simulink model "Sensores"  (R2023b)
settings: Solver=VariableStepAuto  StartTime=0.0  StopTime=10.0  RelTol=1e-3
undefined symbols (not defined in the file): magnitude, Tau_sens_temp, w_n_sens_corr, w_n_sens_pos, zeta_sens
settings Model: Creator=tomas  LastModifiedBy=tomas

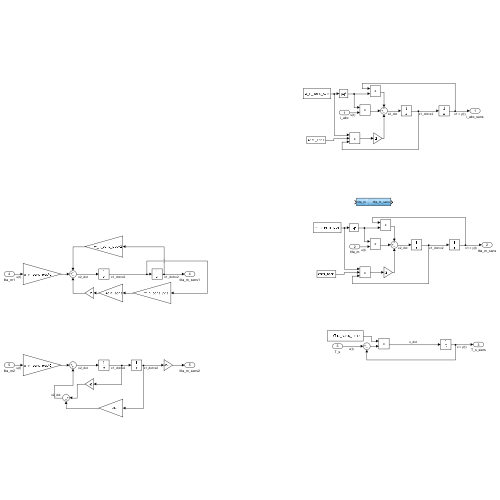
[thumbnail: Simulink's stored preview of the top-level diagram]
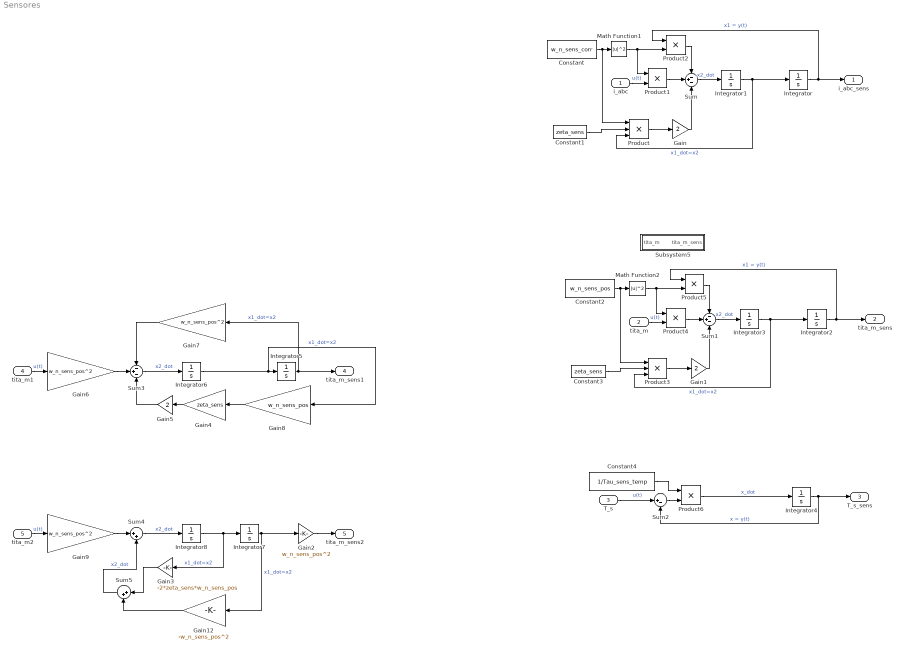
== system Sensores ==
  i_abc : Inport
  tita_m : Inport  Port=2
  T_s : Inport  Port=3
  tita_m1 : Inport  Port=4
  tita_m2 : Inport  Port=5
  Constant : Constant  Value=w_n_sens_corr
  Constant1 : Constant  Value=zeta_sens
  Constant2 : Constant  Value=w_n_sens_pos
  Constant3 : Constant  Value=zeta_sens
  Constant4 : Constant  Value=1/Tau_sens_temp
  Gain : Gain  Gain=2
  Gain1 : Gain  Gain=2
  Gain12 : Gain  Gain=-w_n_sens_pos^2
  Gain{2,6..7,9} (4 alike) : Gain  Gain=w_n_sens_pos^2
  Gain3 : Gain  Gain=-2*zeta_sens*w_n_sens_pos
  Gain4 : Gain  Gain=zeta_sens
  Gain5 : Gain  Gain=2
  Gain8 : Gain  Gain=w_n_sens_pos
  Integrator{,1..8} (9 alike) : Integrator
  Math Function1 : Math  Operator=magnitude^2
  Math Function2 : Math  Operator=magnitude^2
  Product : Product  Inputs=3
  Product{1..2,4..6} (5 alike) : Product
  Product3 : Product  Inputs=3
  Subsystem5 : Subsystem
  Sum : Sum  Inputs=-+-
  Sum1 : Sum  Inputs=-+-
  Sum2 : Sum  Inputs=|+-
  Sum3 : Sum  Inputs=-+-
  Sum4 : Sum  Inputs=|++
  Sum5 : Sum  Inputs=|++
  i_abc_sens : Outport
  tita_m_sens : Outport  Port=2
  T_s_sens : Outport  Port=3
  tita_m_sens1 : Outport  Port=4
  tita_m_sens2 : Outport  Port=5
  wires:
  Integrator/1 -> i_abc_sens/1, Product2/1  "x1 = y(t)"
  Integrator1/1 -> Product/3, Integrator/1  "x1_dot=x2"
  Constant/1 -> Product/1, Math Function1/1
  i_abc/1 -> Product1/2  "u(t)"
  Math Function1/1 -> Product2/2, Product1/1
  Product1/1 -> Sum/2
  Product2/1 -> Sum/1
  Product/1 -> Gain/1
  Gain/1 -> Sum/3
  Sum/1 -> Integrator1/1  "x2_dot"
  Constant1/1 -> Product/2
  Product4/1 -> Sum1/2
  Gain1/1 -> Sum1/3
  Constant2/1 -> Product3/1, Math Function2/1
  tita_m/1 -> Product4/2  "u(t)"
  Product3/1 -> Gain1/1
  Product5/1 -> Sum1/1
  Math Function2/1 -> Product5/2, Product4/1
  Sum1/1 -> Integrator3/1  "x2_dot"
  Constant3/1 -> Product3/2
  Integrator3/1 -> Product3/3, Integrator2/1  "x1_dot=x2"
  Integrator2/1 -> tita_m_sens/1, Product5/1  "x1 = y(t)"
  Integrator4/1 -> Sum2/2, T_s_sens/1  "x = y(t)"
  Product6/1 -> Integrator4/1  "x_dot"
  T_s/1 -> Sum2/1  "u(t)"
  Sum2/1 -> Product6/2
  Constant4/1 -> Product6/1
  tita_m1/1 -> Gain6/1  "u(t)"
  Gain6/1 -> Sum3/2
  Sum3/1 -> Integrator6/1  "x2_dot"
  Integrator6/1 -> Gain8/1, Integrator5/1  "x1_dot=x2"
  Integrator5/1 -> Gain7/1, tita_m_sens1/1  "x1_dot=x2"
  Gain7/1 -> Sum3/1
  Gain5/1 -> Sum3/3
  Gain4/1 -> Gain5/1
  Gain8/1 -> Gain4/1
  Integrator8/1 -> Gain3/1, Integrator7/1  "x1_dot=x2"
  tita_m2/1 -> Gain9/1  "u(t)"
  Sum4/1 -> Integrator8/1  "x2_dot"
  Gain12/1 -> Sum5/2
  Gain3/1 -> Sum5/1
  Sum5/1 -> Sum4/2  "x2_dot"
  Gain9/1 -> Sum4/1
  Integrator7/1 -> Gain12/1, Gain2/1  "x1_dot=x2"
  Gain2/1 -> tita_m_sens2/1

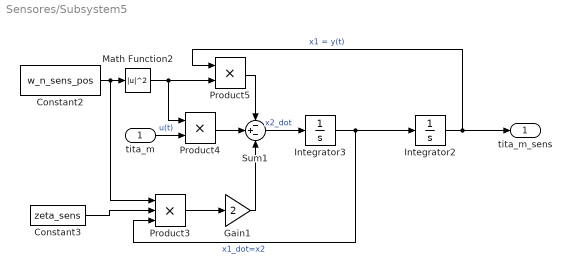
== system Sensores/Subsystem5 ==
  tita_m : Inport
  Constant2 : Constant  Value=w_n_sens_pos
  Constant3 : Constant  Value=zeta_sens
  Gain1 : Gain  Gain=2
  Integrator2 : Integrator
  Integrator3 : Integrator
  Math Function2 : Math  Operator=magnitude^2
  Product3 : Product  Inputs=3
  Product4 : Product
  Product5 : Product
  Sum1 : Sum  Inputs=-+-
  tita_m_sens : Outport
  wires:
  Constant2/1 -> Product3/1, Math Function2/1
  Gain1/1 -> Sum1/3
  Product4/1 -> Sum1/2
  Integrator3/1 -> Product3/3, Integrator2/1  "x1_dot=x2"
  Product3/1 -> Gain1/1
  Constant3/1 -> Product3/2
  Math Function2/1 -> Product5/2, Product4/1
  Product5/1 -> Sum1/1
  tita_m/1 -> Product4/2  "u(t)"
  Sum1/1 -> Integrator3/1  "x2_dot"
  Integrator2/1 -> tita_m_sens/1, Product5/1  "x1 = y(t)"
